simulink model "Option2"  (R2023b)
settings: Solver=FixedStepAuto  StartTime=0.0  StopTime=25  FixedStep=dT  RelTol=1e-3
undefined symbols (not defined in the file): a, Bc, Jc
settings Model: Creator=joshc  LastModifiedBy=huert

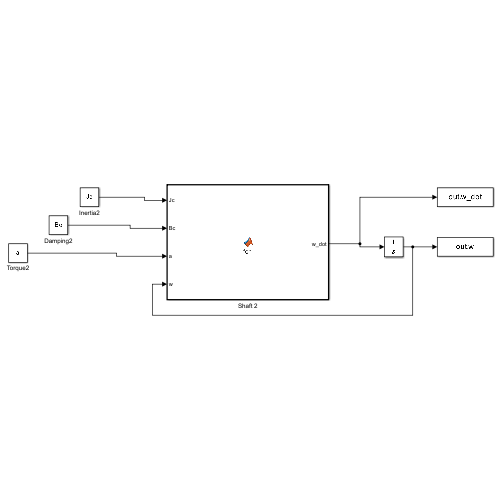
[thumbnail: Simulink's stored preview of the top-level diagram]
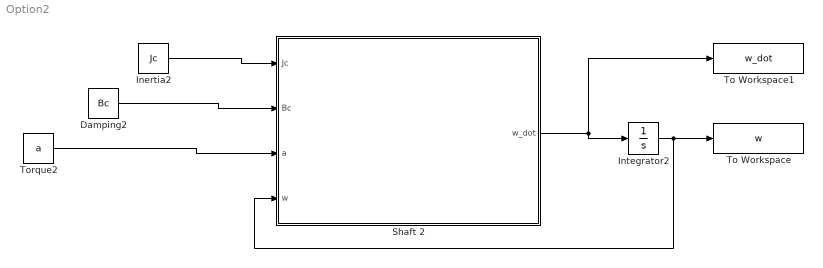
== system Option2 ==
  Damping2 : Constant  Value=Bc
  Inertia2 : Constant  Value=Jc
  Integrator2 : Integrator  UpperSaturationLimit=1000
  Shaft 2 : MATLAB Function  TreatAsAtomicUnit=on
  To Workspace : ToWorkspace  VariableName=w  SaveFormat=Structure With Time  SampleTime=-1
  To Workspace1 : ToWorkspace  VariableName=w_dot  SaveFormat=Structure With Time  SampleTime=-1
  Torque2 : Constant  Value=a
  wires:
  Integrator2/1 -> Shaft 2/4(w), To Workspace/1
  Shaft 2/1(w_dot) -> To Workspace1/1, Integrator2/1
  Torque2/1 -> Shaft 2/3(a)
  Damping2/1 -> Shaft 2/2(Bc)
  Inertia2/1 -> Shaft 2/1(Jc)

== matlab function Option2/Shaft 2 ==
  data: Jc input; w_dot output; Bc input; a input; w input
function w_dot = fcn(Jc, Bc, a, w)

w_dot = (1/Jc)*(a - Bc*w);

end
